simulink model "delay_based_echo"  (R2020b)
settings: Solver=FixedStepDiscrete  StartTime=0.0  StopTime=stopTime  RelTol=1e-3
InitFcn:
  | initCallback
StopFcn:
  | stopCallback
undefined symbols (not defined in the file or in its folder): config
settings Model: Creator=Ross  LastModifiedBy=conno
settings SolverCC: MinimalZcImpactIntegration=on
settings DataIOCC: ReturnWorkspaceOutputs=off
settings OptimizationCC: DefaultParameterBehavior=Inlined
settings DebuggingCC: ReadBeforeWriteMsg=DisableAll  WriteAfterWriteMsg=DisableAll  WriteAfterReadMsg=DisableAll  AlgebraicLoopMsg=error  MultiTaskDSMMsg=none  SingleTaskRateTransMsg=error  PregeneratedLibrarySubsystemCodeDiagnostic=none  ArithmeticOperatorsInVariantConditions=warning
settings HardwareCC: ProdBitPerPointer=32  ProdBitPerSizeT=32  ProdBitPerPtrDiffT=32  ProdLargestAtomicFloat=None  ProdIntDivRoundTo=Undefined  ProdEndianess=Unspecified  ProdWordSize=32  ProdHWDeviceType=ASIC/FPGA->ASIC/FPGA  TargetBitPerPointer=64  TargetBitPerSizeT=64  TargetBitPerPtrDiffT=64  TargetLongLongMode=on  TargetIntDivRoundTo=Zero  TargetEndianess=LittleEndian  TargetWordSize=64  TargetHWDeviceType=Custom Processor->MATLAB Host Computer  ProdEqTarget=off
settings ModelReferenceCC: UpdateModelReferenceTargets=IfOutOfDate
settings SFSimCC: SFSimEcho=off  SimUseLocalCustomCode=off  CustomCodeUndefinedFunction=UseInterfaceOnly
settings RTWCC: RTWUseLocalCustomCode=off

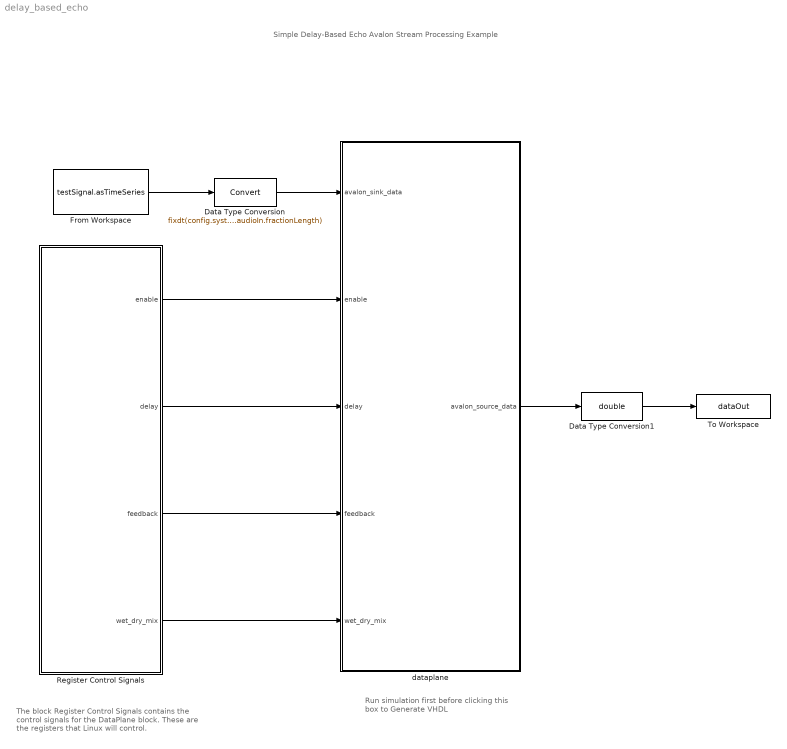
== system delay_based_echo ==
  note: Simple Delay-Based Echo
      | Avalon Stream Processing Example
  note: Run simulation first
      | before clicking this box to
      | Generate VHDL
  note: The block Register Control Signals contains
      | the control signals for the DataPlane block.
      | These are the registers that Linux will control.
  Data Type Conversion : DataTypeConversion  OutDataTypeStr=fixdt(config.system.audioIn.signed, config.system.audioIn.wordLength, config.system.audioIn.fractionLength)
  Data Type Conversion1 : DataTypeConversion  OutDataTypeStr=double
  From Workspace : FromWorkspace  VariableName=testSignal.asTimeSeries  SampleTime=1 / config.system.sampleClockFrequency  OutputAfterFinalValue=Setting to zero
  Register Control Signals : Subsystem
  To Workspace : ToWorkspace  VariableName=dataOut  SaveFormat=Timeseries  SampleTime=-1
  dataplane : Subsystem  TreatAsAtomicUnit=on
  wires:
  dataplane/1(avalon_source_data) -> Data Type Conversion1/1
  Register Control Signals/2(delay) -> dataplane/3(delay)
  Register Control Signals/1(enable) -> dataplane/2(enable)
  Register Control Signals/4(wet_dry_mix) -> dataplane/5(wet_dry_mix)
  Register Control Signals/3(feedback) -> dataplane/4(feedback)
  From Workspace/1 -> Data Type Conversion/1
  Data Type Conversion/1 -> dataplane/1(avalon_sink_data)
  Data Type Conversion1/1 -> To Workspace/1

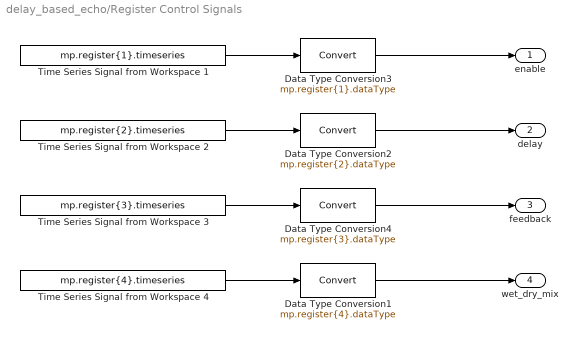
== system delay_based_echo/Register Control Signals ==
  Data Type Conversion1 : DataTypeConversion  OutDataTypeStr=mp.register{4}.dataType
  Data Type Conversion2 : DataTypeConversion  OutDataTypeStr=mp.register{2}.dataType
  Data Type Conversion3 : DataTypeConversion  OutDataTypeStr=mp.register{1}.dataType
  Data Type Conversion4 : DataTypeConversion  OutDataTypeStr=mp.register{3}.dataType
  Time Series Signal from Workspace 1 : FromWorkspace  VariableName=mp.register{1}.timeseries  OutDataTypeStr=double  SampleTime=1 / config.system.sampleClockFrequency
  Time Series Signal from Workspace 2 : FromWorkspace  VariableName=mp.register{2}.timeseries  OutDataTypeStr=double  SampleTime=1 / config.system.sampleClockFrequency
  Time Series Signal from Workspace 3 : FromWorkspace  VariableName=mp.register{3}.timeseries  OutDataTypeStr=double  SampleTime=1 / config.system.sampleClockFrequency
  Time Series Signal from Workspace 4 : FromWorkspace  VariableName=mp.register{4}.timeseries  OutDataTypeStr=double  SampleTime=1 / config.system.sampleClockFrequency
  enable : Outport  VectorParamsAs1DForOutWhenUnconnected=off
  delay : Outport  Port=2  VectorParamsAs1DForOutWhenUnconnected=off
  feedback : Outport  Port=3  VectorParamsAs1DForOutWhenUnconnected=off
  wet_dry_mix : Outport  Port=4  VectorParamsAs1DForOutWhenUnconnected=off
  wires:
  Time Series Signal from Workspace 2/1 -> Data Type Conversion2/1
  Data Type Conversion2/1 -> delay/1
  Time Series Signal from Workspace 1/1 -> Data Type Conversion3/1
  Data Type Conversion3/1 -> enable/1
  Time Series Signal from Workspace 4/1 -> Data Type Conversion1/1
  Data Type Conversion1/1 -> wet_dry_mix/1
  Data Type Conversion4/1 -> feedback/1
  Time Series Signal from Workspace 3/1 -> Data Type Conversion4/1

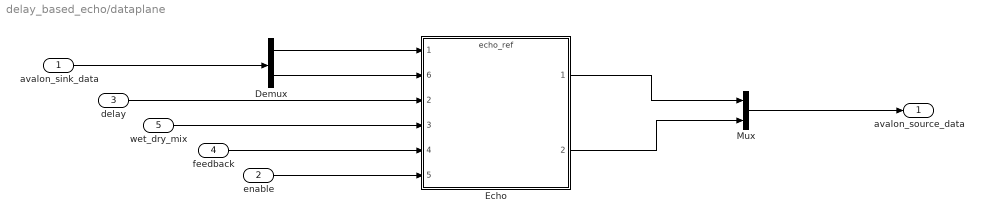
== system delay_based_echo/dataplane ==
  avalon_sink_data : Inport
  enable : Inport  Port=2
  delay : Inport  Port=3
  feedback : Inport  Port=4
  wet_dry_mix : Inport  Port=5
  Demux : Demux  Outputs=2
  Echo : ModelReference  ModelNameDialog=echo_ref  SimulationMode=Normal  ModelReferenceVersion=1.165
      settings: PortSchema="{\"entries\":[{\"content\":{\"sides\":[{\"content\":{\"connectorIds\":[\"In1\",\"In6\",\"In2\",\"In3\",\"In4\",\"In5\"]},\"type\":\"ConnectorPlacement.EquallySpacedRectSide\",\"uuid\":\"e306e1ad-d1b8-4582-952d-4c4191a99a81\"},{\"content\":{\"connectorIds\":[\"Out1\",\"Out2\"],\"side\":\"RIGHT\"},\"type\":\"ConnectorPlacement.EquallySpacedRectSide\",\"uuid\":\"8133f08a-39d0-44da-b52e-b96b1c72783c\"},{\"content\":{\"connectorIds\":[],\"side\":\"TOP\"},\"type\":\"ConnectorPlacement.EquallySpacedRectSide\",\"uuid\":\"327e31c7-8f91-4124-82a4-b2c62ce56765\"},{\"content\":{\"connectorIds\":[],\"side\":\"HIDDEN\"},\"type\":\"ConnectorPlacement.EquallySpacedRectSide\",\"uuid\":\"f85fe833-603d-4d04-9a61-60dde0930239\"}]},\"type\":\"ConnectorPlacement.EquallySpacedConnector\",\"uuid\":\"c6b2a458-4634-4ce8-98bc-50a2a0ff1bc4\"}],\"packageUris\":[\"http://schema.mathworks.com/mf0/Connector/R2020b\"],\"version\":\"1.0\"}"
  Mux : Mux  Inputs=2
  avalon_source_data : Outport  VectorParamsAs1DForOutWhenUnconnected=off
  wires:
  avalon_sink_data/1 -> Demux/1
  delay/1 -> Echo/2
  wet_dry_mix/1 -> Echo/3
  feedback/1 -> Echo/4
  enable/1 -> Echo/5
  Demux/1 -> Echo/1
  Demux/2 -> Echo/6
  Echo/1 -> Mux/1
  Echo/2 -> Mux/2
  Mux/1 -> avalon_source_data/1
